simulink model "Rate_Modulation_2"  (R2023a)
settings: Solver=VariableStepAuto  StartTime=0.0  StopTime=100  RelTol=1e-3
model workspace (MAT data in the model file):
  Acc_threshold = Simulink.Parameter
  Acc_threshold.Value = 10
  Acc_threshold.Description = 'minimo valore dell''accelerometro per cui considero paziente in attività'
  Acc_threshold.DataType = 'auto'
  Acc_threshold.Complexity = 'real'
  Acc_threshold.Dimensions = [1 1]
  Activity_response_factor = Simulink.Parameter
  Activity_response_factor.Value = 0.4
  Activity_response_factor.Description = '0<activity response factor<1
    | 
    | max activity setup: activity response factor=1, cioè si raggiunge solo alla massima capacità del sensore il valore MSR_TOP
    | '
  Activity_response_factor.DataType = 'auto'
  Activity_response_factor.Complexity = 'real'
  Activity_response_factor.Dimensions = [1 1]
  Baseline = Simulink.Parameter
  Baseline.Value = 144
  Baseline.Description = 'respiratory rate (average:12) * tidal volume (average:12) in the person
    | -> varies depending on height age gender'
  Baseline.DataType = 'auto'
  Baseline.Complexity = 'real'
  Baseline.Dimensions = [1 1]
  LRL = Simulink.Parameter
  LRL.Value = 60
  LRL.Description = 'Lowest Rate Level'
  LRL.DataType = 'auto'
  LRL.Complexity = 'real'
  LRL.Dimensions = [1 1]
  MSR = Simulink.Parameter
  MSR.Value = 150
  MSR.Description = 'Max Stimulated Rate'
  MSR.DataType = 'auto'
  MSR.Complexity = 'real'
  MSR.Dimensions = [1 1]
  MSR_TOP = Simulink.Parameter
  MSR_TOP.Value = 220
  MSR_TOP.Description = 'max msr: quello con cui faccio le curve, non l''effettivo limite
    | 
    | oss: LRL non ha questa distinzione perchè tendenzialmente è sempre lo stesso'
  MSR_TOP.DataType = 'auto'
  MSR_TOP.Complexity = 'real'
  MSR_TOP.Dimensions = [1 1]
  Metabolic_response_factor = Simulink.Parameter
  Metabolic_response_factor.Value = 0.8
  Metabolic_response_factor.Description = '0<Metabolic_response_factor<1
    | 
    | max metabolic setup: Metabolic_response_factor=1, cioè si raggiunge solo alla massima capacità del sensore il valore MSR_TOP
    | '
  Metabolic_response_factor.DataType = 'auto'
  Metabolic_response_factor.Complexity = 'real'
  Metabolic_response_factor.Dimensions = [1 1]
  Plateau = Simulink.Parameter
  Plateau.Value = 90
  Plateau.Description = '90-95'
  Plateau.DataType = 'auto'
  Plateau.Complexity = 'real'
  Plateau.Dimensions = [1 1]
  Rate_modulation_type = Simulink.Parameter
  Rate_modulation_type.Value = 3
  Rate_modulation_type.Description = '1: integrazione1
    | 2: integrazione2
    | 3: solo acc
    | 4: solo mv'
  Rate_modulation_type.DataType = 'auto'
  Rate_modulation_type.Complexity = 'real'
  Rate_modulation_type.Dimensions = [1 1]
  Reaction_time = 10
  VT_BPM = Simulink.Parameter
  VT_BPM.Value = 156
  VT_BPM.Description = 'battiti a cui corrisponde MV threshold dato il response factor detereminato da MSR e LRL
    | con Ventilatory_Threshold = 60 -> 156 (60-220)
    | '
  VT_BPM.DataType = 'auto'
  VT_BPM.Complexity = 'real'
  VT_BPM.Dimensions = [1 1]
  Ventilatory_Threshold = Simulink.Parameter
  Ventilatory_Threshold.Value = 60
  Ventilatory_Threshold.DataType = 'auto'
  Ventilatory_Threshold.Complexity = 'real'
  Ventilatory_Threshold.Dimensions = [1 1]
  Ventilatory_threshold_response = Simulink.Parameter
  Ventilatory_threshold_response.Value = 0.8
  Ventilatory_threshold_response.Description = '1: OFF
    | 0<Ventilatory_threshold_response<1 '
  Ventilatory_threshold_response.DataType = 'auto'
  Ventilatory_threshold_response.Complexity = 'real'
  Ventilatory_threshold_response.Dimensions = [1 1]
undefined symbols (not defined in the file or in its folder): MAX_MV
libraries: SignalEditorBlockLib x1, dspstat3 x1
settings Model: Creator=fican  LastModifiedBy=fican
settings DebuggingCC: UnconnectedInputMsg=warning  UnconnectedOutputMsg=warning  UnconnectedLineMsg=warning
settings ModelReferenceCC: EnableRefExpFcnMdlSchedulingChecks=on
settings RTWCC: DLArmComputeVersion=19.05

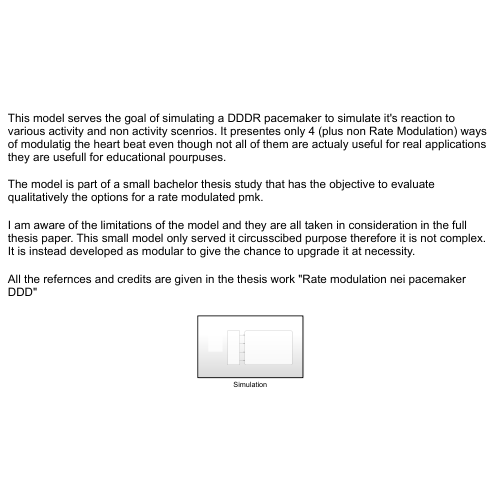
[thumbnail: Simulink's stored preview of the top-level diagram]
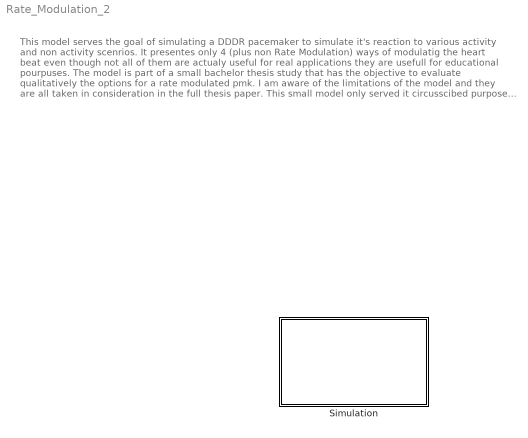
== system Rate_Modulation_2 ==
  note: This model serves the goal of simulating a DDDR pacemaker to simulate it's reaction to various activity and non activity scenrios. It presentes only 4 (plus non Rate Modulation) ways of modulatig the heart beat even though not all of them are actualy useful for real applications they are usefull for educational pourpuses.
      |
      | The model is part of a small bachelor thesis study that has the objective to evaluate qualitatively the options for a rate modulated pmk.
      |
      | I am aware of the limitations of the model and they are all taken in consideration in the full thesis paper. This small model only served it circusscibed purpose therefore it is not complex. It is instead developed as modular to give the chance to upgrade it at necessity.
      |
      | All the refernces and credits are given in the thesis work "Rate modulation nei pacemaker DDD"
  Simulation : Subsystem

== system Rate_Modulation_2/Simulation ==
  note: This stateflow subsystem is the heart of the model
      |
      |
      | sorry for the word play, i had to do it.
  note: This block gives in input simple scenarios created specifally to evaluate the model behaviour in some circustances. It has already a list of some geeric conditions and some limit ones.
      |
      | The only sensors taken for this model are an accelerometer as activity sensor and a minute ventilation as a metabolic sensor.
  Input scenario : SignalEditorBlockLib/Signal Editor  FileName=Scenario2.mat  ActiveScenario=Esercizio  ActiveSignal=Atrium_0  IsBus=off  OutputBusObjectStr=Bus: BusObject  SampleTime=0.001  Interpolate=off  ZeroCross=off  OutputAfterFinalValue=Setting to zero  Unit=inherit  PreserveSignalName=on  ApplySigPropsToAllScenarios=on
  Pacemaker : Stateflow chart  TreatAsAtomicUnit=on
  wires:
  Input scenario/1 -> Pacemaker/1(Atrium)
  Input scenario/3 -> Pacemaker/3(acc_percent)
  Input scenario/2 -> Pacemaker/2(Ventricle)
  Input scenario/4 -> Pacemaker/4(mv_percent)

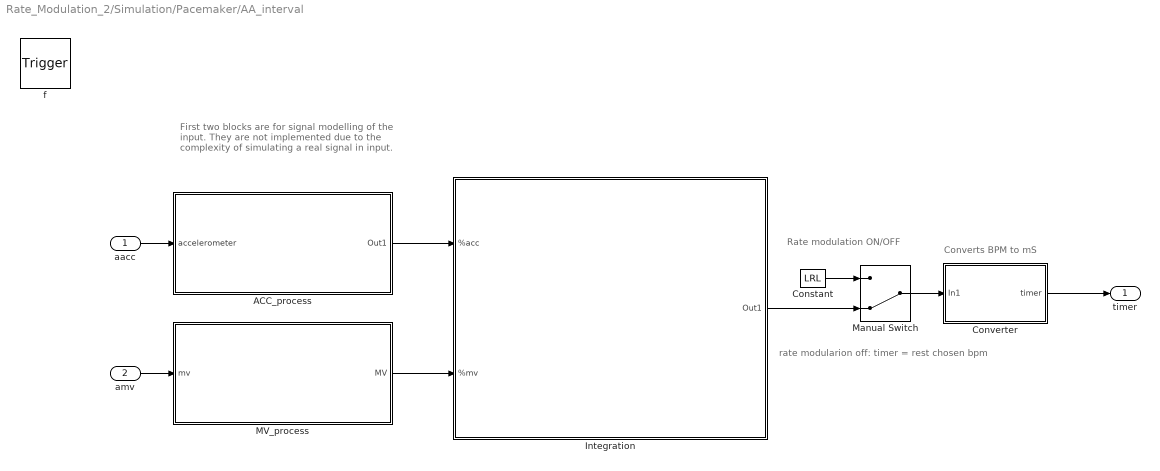
== system Rate_Modulation_2/Simulation/Pacemaker/AA_interval ==
  note: Rate modulation ON/OFF
  note: First two blocks are for signal modelling of the input. They are not implemented due to the complexity of simulating a real signal in input.
  note: Converts BPM to mS
  note: rate modularion off: timer = rest chosen bpm
  aacc : Inport  OutDataTypeStr=double  Unit=1  PortDimensions=1
  amv : Inport  Port=2  OutDataTypeStr=double  Unit=1  PortDimensions=1
  f : TriggerPort  TriggerType=function-call  VariantControl=(inherit)
      settings: CopyFcn=Stateflow.SLINSF.SimulinkMan.removeBlockPreDeleteFcn  PreDeleteFcn=Stateflow.SLINSF.SimulinkMan.unsafePredeleteFcn
  ACC_process : Subsystem
  Constant : Constant  Value=LRL
  Converter : Subsystem
  Integration : Subsystem
  MV_process : Subsystem
  Manual Switch : ManualSwitch  CurrentSetting=0
  timer : Outport
  wires:
  Constant/1 -> Manual Switch/1
  Integration/1(Out1) -> Manual Switch/2
  Converter/1(timer) -> timer/1
  Manual Switch/1 -> Converter/1(In1)
  aacc/1 -> ACC_process/1(accelerometer)
  amv/1 -> MV_process/1(mv)
  ACC_process/1(Out1) -> Integration/1(%acc)
  MV_process/1(MV) -> Integration/2(%mv)

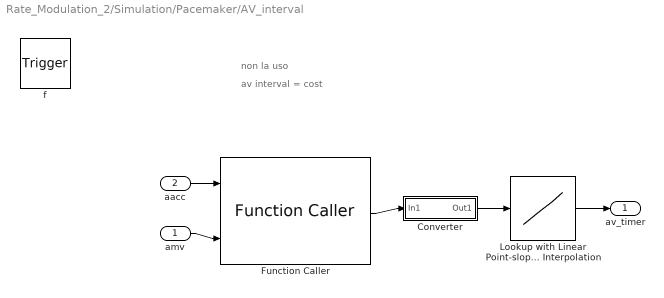
== system Rate_Modulation_2/Simulation/Pacemaker/AV_interval ==
  note: av interval = cost
  note: non la uso
  amv : Inport  OutDataTypeStr=int64  PortDimensions=1
      settings: VarSizeSig=Yes
  aacc : Inport  Port=2  OutDataTypeStr=double  Unit=1  PortDimensions=1
      settings: SignalType=complex
  f : TriggerPort  TriggerType=function-call  VariantControl=(inherit)
      settings: CopyFcn=Stateflow.SLINSF.SimulinkMan.removeBlockPreDeleteFcn  PreDeleteFcn=Stateflow.SLINSF.SimulinkMan.unsafePredeleteFcn
  Converter : Subsystem
  Function Caller : FunctionCaller  FunctionPrototype=timer = AA_interval(aacc,amv)  InputArgumentSpecifications=<Enter example>  OutputArgumentSpecifications=<Enter example>
  Lookup with Linear Point-slope Interpolation : Lookup_n-D  NumberOfTableDimensions=1  BreakpointsForDimension1=[LRL 120]  Table=[175 135]  InternalRulePriority=Speed  RndMeth=Simplest
  av_timer : Outport
  wires:
  aacc/1 -> Function Caller/1
  amv/1 -> Function Caller/2
  Lookup with Linear Point-slope Interpolation/1 -> av_timer/1
  Function Caller/1 -> Converter/1(In1)
  Converter/1(Out1) -> Lookup with Linear Point-slope Interpolation/1

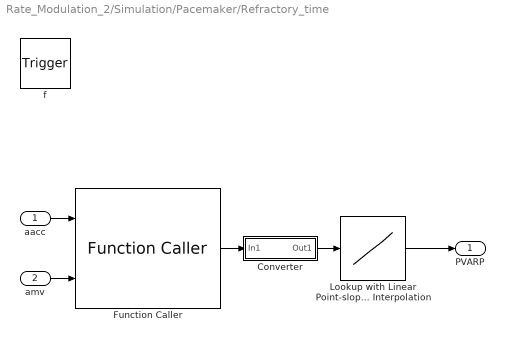
== system Rate_Modulation_2/Simulation/Pacemaker/Refractory_time ==
  aacc : Inport  OutDataTypeStr=double  PortDimensions=1
  amv : Inport  Port=2  OutDataTypeStr=double  PortDimensions=1
  f : TriggerPort  TriggerType=function-call  VariantControl=(inherit)
      settings: CopyFcn=Stateflow.SLINSF.SimulinkMan.removeBlockPreDeleteFcn  PreDeleteFcn=Stateflow.SLINSF.SimulinkMan.unsafePredeleteFcn
  Converter : Subsystem
  Function Caller : FunctionCaller  FunctionPrototype=timer = AA_interval(aacc,amv)  InputArgumentSpecifications=<Enter example>  OutputArgumentSpecifications=<Enter example>
  Lookup with Linear Point-slope Interpolation : Lookup_n-D  NumberOfTableDimensions=1  BreakpointsForDimension1=[LRL 120]  Table=[400 370]  InternalRulePriority=Speed  RndMeth=Simplest
  PVARP : Outport
  wires:
  aacc/1 -> Function Caller/1
  amv/1 -> Function Caller/2
  Function Caller/1 -> Converter/1(In1)
  Converter/1(Out1) -> Lookup with Linear Point-slope Interpolation/1
  Lookup with Linear Point-slope Interpolation/1 -> PVARP/1

== system Rate_Modulation_2/Simulation/Pacemaker/AA_interval/ACC_process ==
  note: The idea here was just to convert the volt signal to a 0-100 value that indicates how much activity is done by the patient. In this model the processing of the signal is not present.
      |
      | It is only present the gain that allows the 'doctor' to regulate the response to activity factor.
      |
      | The simplest way in wich i would have inplemented the signal processing would have been to convert the volt input into a frequency value (considering the smallest period of the oscillatinf signal). This value would have been interpoled beween 0-100 (the actual value input that i'm considering project standing) with the lowest (probably respiratory rate and not zero) and maximum frequency i would have expected from my sensor.
  accelerometer : Inport
  Gain : Gain  Gain=Activity_response_factor
  Out1 : Outport
  wires:
  Gain/1 -> Out1/1
  accelerometer/1 -> Gain/1

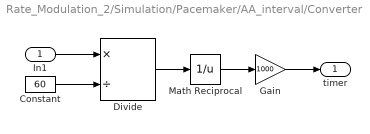
== system Rate_Modulation_2/Simulation/Pacemaker/AA_interval/Converter ==
  In1 : Inport
  Constant : Constant  Value=60
  Divide : Product  Inputs=*/
  Gain : Gain  Gain=1000
  Math Reciprocal : Math  Operator=reciprocal  SignedPower=on
  timer : Outport
  wires:
  In1/1 -> Divide/1
  Constant/1 -> Divide/2
  Divide/1 -> Math Reciprocal/1
  Math Reciprocal/1 -> Gain/1
  Gain/1 -> timer/1

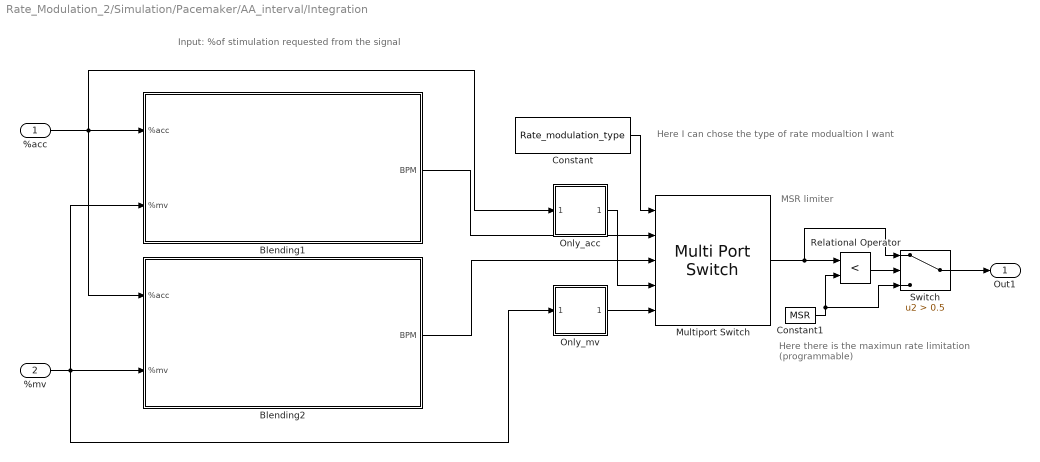
== system Rate_Modulation_2/Simulation/Pacemaker/AA_interval/Integration ==
  note: MSR limiter
  note: Here there is the maximun rate limitation (programmable)
  note: Input: %of stimulation requested from the signal
  note: Here I can chose the type of rate modualtion I want
  %acc : Inport
  %mv : Inport  Port=2
  Blending1 : Subsystem
  Blending2 : Subsystem
  Constant : Constant  Value=Rate_modulation_type
  Constant1 : Constant  Value=MSR
  Multiport Switch : MultiPortSwitch  Inputs=4  DataPortIndices={1,2,3,0}  SaturateOnIntegerOverflow=off  InputSameDT=off
  Only_acc : Subsystem
  Only_mv : Subsystem
  Relational Operator : RelationalOperator  Operator=<  OutDataTypeStr=boolean  RndMeth=Simplest  InputSameDT=off
  Switch : Switch  Criteria=u2 > Threshold  Threshold=0.5  RndMeth=Round  SaturateOnIntegerOverflow=off  InputSameDT=off
  Out1 : Outport
  wires:
  Constant/1 -> Multiport Switch/1
  %acc/1 -> Only_acc/1(%acc), Blending1/1(%acc), Blending2/1(%acc)
  %mv/1 -> Blending2/2(%mv), Only_mv/1(%mv), Blending1/2(%mv)
  Only_acc/1(Out1) -> Multiport Switch/4
  Only_mv/1(Out1) -> Multiport Switch/5
  Blending1/1(BPM) -> Multiport Switch/2
  Blending2/1(BPM) -> Multiport Switch/3
  Multiport Switch/1 -> Switch/1, Relational Operator/1
  Constant1/1 -> Relational Operator/2, Switch/3
  Relational Operator/1 -> Switch/2
  Switch/1 -> Out1/1

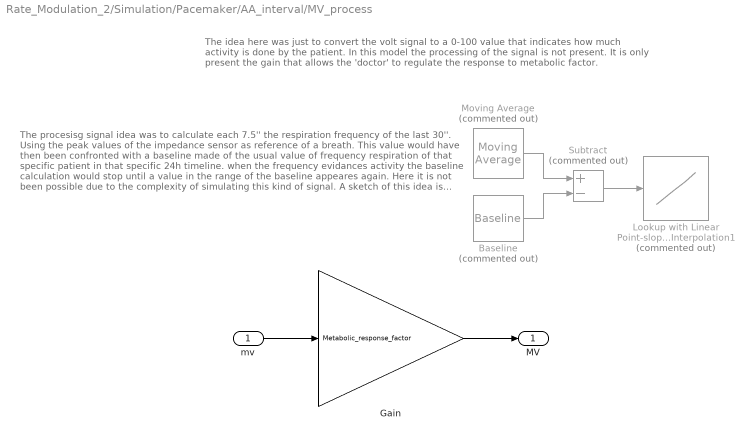
== system Rate_Modulation_2/Simulation/Pacemaker/AA_interval/MV_process ==
  note: The procesisg signal idea was to calculate each 7.5'' the respiration frequency of the last 30''. Using the peak values of the impedance sensor as reference of a breath. This value would have then been confronted with a baseline made of the usual value of frequency respiration of that specific patient in that specific 24h timeline. when the frequency evidances activity the baseline calculation would stop until a value in the range of the baseline appeares again.
      |
      | Here it is not been possible due to the complexity of simulating this kind of signal. A sketch of this idea is present here as a comment.
  note: The idea here was just to convert the volt signal to a 0-100 value that indicates how much activity is done by the patient. In this model the processing of the signal is not present.
      |
      | It is only present the gain that allows the 'doctor' to regulate the response to metabolic factor.
  mv : Inport
  Baseline : Constant  Commented=on  Value=Baseline
  Gain : Gain  Gain=Metabolic_response_factor
  Lookup with Linear Point-slope Interpolation1 : Lookup_n-D  Commented=on  NumberOfTableDimensions=1  BreakpointsForDimension1=[0 MAX_MV]  Table=[0 100]  InternalRulePriority=Speed  RndMeth=Simplest
  Moving Average : dspstat3/Moving Average  Commented=on  Method=Sliding window  ForgettingFactorPort=off  SpecifyWindowLength=on  WindowLength=30  OverlapLength=29  AllowArbitraryInputLength=off  ForgettingFactor=0.9  SimulateUsing=Code generation
  Subtract : Sum  Commented=on  Inputs=+-
  MV : Outport
  wires:
  Baseline/1 -> Subtract/2
  Moving Average/1 -> Subtract/1
  Subtract/1 -> Lookup with Linear Point-slope Interpolation1/1
  mv/1 -> Gain/1
  Gain/1 -> MV/1

== system Rate_Modulation_2/Simulation/Pacemaker/AV_interval/Converter ==
  In1 : Inport
  Gain : Gain  Gain=0.001
  Gain1 : Gain  Gain=60
  Math Reciprocal : Math  Operator=reciprocal  SignedPower=on
  Out1 : Outport
  wires:
  Gain/1 -> Math Reciprocal/1
  In1/1 -> Gain/1
  Math Reciprocal/1 -> Gain1/1
  Gain1/1 -> Out1/1

== system Rate_Modulation_2/Simulation/Pacemaker/Refractory_time/Converter ==
  In1 : Inport
  Gain : Gain  Gain=0,001
  Gain1 : Gain  Gain=60
  Math Reciprocal : Math  Operator=reciprocal  SignedPower=on
  Out1 : Outport
  wires:
  Gain/1 -> Math Reciprocal/1
  In1/1 -> Gain/1
  Math Reciprocal/1 -> Gain1/1
  Gain1/1 -> Out1/1

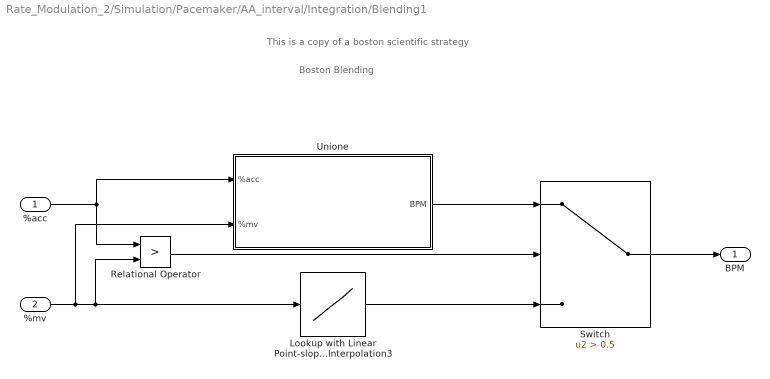
== system Rate_Modulation_2/Simulation/Pacemaker/AA_interval/Integration/Blending1 ==
  note: This is a copy of a boston scientific strategy
  note: Boston Blending
  %acc : Inport
  %mv : Inport  Port=2
  Lookup with Linear Point-slope Interpolation3 : Lookup_n-D  NumberOfTableDimensions=1  BreakpointsForDimension1=[0 100]  Table=[LRL MSR_TOP]  InternalRulePriority=Speed  RndMeth=Simplest
  Relational Operator : RelationalOperator  Operator=>  OutDataTypeStr=boolean  RndMeth=Simplest  InputSameDT=off
  Switch : Switch  Criteria=u2 > Threshold  Threshold=0.5  SaturateOnIntegerOverflow=off  InputSameDT=off
  Unione : Subsystem
  BPM : Outport
  wires:
  %acc/1 -> Unione/1(%acc), Relational Operator/1
  %mv/1 -> Relational Operator/2, Lookup with Linear Point-slope Interpolation3/1, Unione/2(%mv)
  Relational Operator/1 -> Switch/2
  Switch/1 -> BPM/1
  Unione/1(BPM) -> Switch/1
  Lookup with Linear Point-slope Interpolation3/1 -> Switch/3

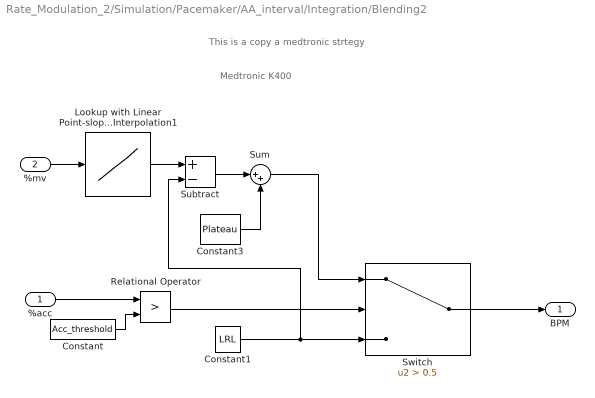
== system Rate_Modulation_2/Simulation/Pacemaker/AA_interval/Integration/Blending2 ==
  note: This is a copy a medtronic strtegy
  note: Medtronic K400
  %acc : Inport
  %mv : Inport  Port=2
  Constant : Constant  Value=Acc_threshold
  Constant1 : Constant  Value=LRL
  Constant3 : Constant  Value=Plateau
  Lookup with Linear Point-slope Interpolation1 : Lookup_n-D  NumberOfTableDimensions=1  BreakpointsForDimension1=[0 100]  Table=[LRL MSR_TOP]  InternalRulePriority=Speed  RndMeth=Simplest
  Relational Operator : RelationalOperator  Operator=>  OutDataTypeStr=boolean  RndMeth=Simplest  InputSameDT=off
  Subtract : Sum  Inputs=+-
  Sum : Sum  Inputs=|++
  Switch : Switch  Criteria=u2 > Threshold  Threshold=0.5  SaturateOnIntegerOverflow=off  InputSameDT=off
  BPM : Outport
  wires:
  %acc/1 -> Relational Operator/1
  Constant/1 -> Relational Operator/2
  Relational Operator/1 -> Switch/2
  Constant1/1 -> Subtract/2, Switch/3
  Lookup with Linear Point-slope Interpolation1/1 -> Subtract/1
  Subtract/1 -> Sum/1
  Constant3/1 -> Sum/2
  %mv/1 -> Lookup with Linear Point-slope Interpolation1/1
  Sum/1 -> Switch/1
  Switch/1 -> BPM/1

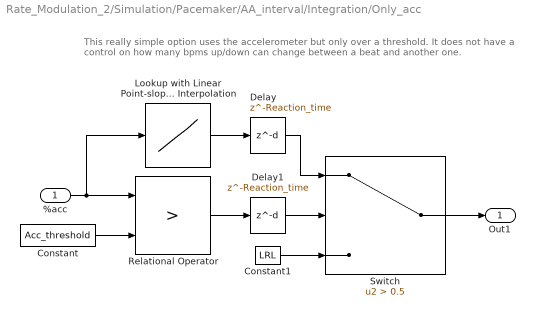
== system Rate_Modulation_2/Simulation/Pacemaker/AA_interval/Integration/Only_acc ==
  note: This really simple option uses the accelerometer but only over a threshold. It does not have a control on how many bpms up/down can change between a beat and another one.
  %acc : Inport
  Constant : Constant  Value=Acc_threshold
  Constant1 : Constant  Value=LRL
  Delay : Delay  DelayLength=Reaction_time
  Delay1 : Delay  DelayLength=Reaction_time
  Lookup with Linear Point-slope Interpolation : Lookup_n-D  NumberOfTableDimensions=1  BreakpointsForDimension1=[Acc_threshold 100+Acc_threshold]  Table=[LRL MSR_TOP]  InternalRulePriority=Speed  RndMeth=Simplest
  Relational Operator : RelationalOperator  Operator=>  OutDataTypeStr=boolean  ZeroCross=off  RndMeth=Simplest  InputSameDT=off
  Switch : Switch  Criteria=u2 > Threshold  Threshold=0.5  OutDataTypeStr=double  SaturateOnIntegerOverflow=off  InputSameDT=off
  Out1 : Outport
  wires:
  Relational Operator/1 -> Delay1/1
  Constant/1 -> Relational Operator/2
  %acc/1 -> Lookup with Linear Point-slope Interpolation/1, Relational Operator/1
  Constant1/1 -> Switch/3
  Delay1/1 -> Switch/2
  Lookup with Linear Point-slope Interpolation/1 -> Delay/1
  Delay/1 -> Switch/1
  Switch/1 -> Out1/1

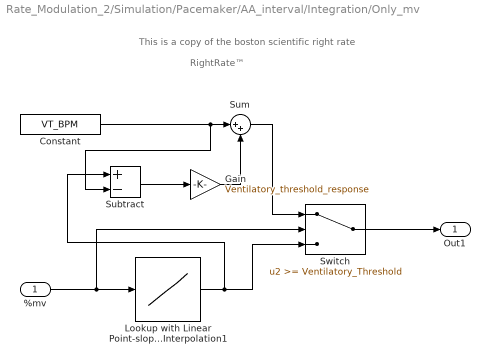
== system Rate_Modulation_2/Simulation/Pacemaker/AA_interval/Integration/Only_mv ==
  note: This is a copy of the boston scientific right rate
  note: RightRate™
  %mv : Inport
  Constant : Constant  Value=VT_BPM
  Gain : Gain  Gain=Ventilatory_threshold_response
  Lookup with Linear Point-slope Interpolation1 : Lookup_n-D  NumberOfTableDimensions=1  BreakpointsForDimension1=[0 100]  Table=[LRL MSR_TOP]  InternalRulePriority=Speed  RndMeth=Simplest
  Subtract : Sum  Inputs=+-
  Sum : Sum  Inputs=|++
  Switch : Switch  Threshold=Ventilatory_Threshold  SaturateOnIntegerOverflow=off  InputSameDT=off
  Out1 : Outport
  wires:
  %mv/1 -> Switch/2, Lookup with Linear Point-slope Interpolation1/1
  Lookup with Linear Point-slope Interpolation1/1 -> Subtract/1, Switch/3
  Switch/1 -> Out1/1
  Constant/1 -> Subtract/2, Sum/1
  Gain/1 -> Sum/2
  Sum/1 -> Switch/1
  Subtract/1 -> Gain/1

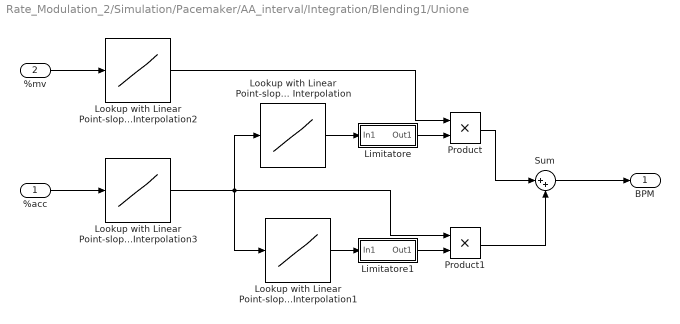
== system Rate_Modulation_2/Simulation/Pacemaker/AA_interval/Integration/Blending1/Unione ==
  %acc : Inport
  %mv : Inport  Port=2
  Limitatore : Subsystem
  Limitatore1 : Subsystem
  Lookup with Linear Point-slope Interpolation : Lookup_n-D  NumberOfTableDimensions=1  BreakpointsForDimension1=[LRL MSR_TOP]  Table=[0.2 0.6]  InternalRulePriority=Speed  RndMeth=Simplest
  Lookup with Linear Point-slope Interpolation1 : Lookup_n-D  NumberOfTableDimensions=1  BreakpointsForDimension1=[LRL MSR_TOP]  Table=[0.8 0.4]  InternalRulePriority=Speed  RndMeth=Simplest
  Lookup with Linear Point-slope Interpolation2 : Lookup_n-D  NumberOfTableDimensions=1  BreakpointsForDimension1=[0 100]  Table=[LRL MSR_TOP]  InternalRulePriority=Speed  RndMeth=Simplest
  Lookup with Linear Point-slope Interpolation3 : Lookup_n-D  NumberOfTableDimensions=1  BreakpointsForDimension1=[0 100]  Table=[LRL MSR_TOP]  InternalRulePriority=Speed  RndMeth=Simplest
  Product : Product
  Product1 : Product
  Sum : Sum  Inputs=|++
  BPM : Outport
  wires:
  %acc/1 -> Lookup with Linear Point-slope Interpolation3/1
  %mv/1 -> Lookup with Linear Point-slope Interpolation2/1
  Product/1 -> Sum/1
  Product1/1 -> Sum/2
  Lookup with Linear Point-slope Interpolation2/1 -> Product/1
  Lookup with Linear Point-slope Interpolation3/1 -> Lookup with Linear Point-slope Interpolation1/1, Product1/1, Lookup with Linear Point-slope Interpolation/1
  Sum/1 -> BPM/1
  Lookup with Linear Point-slope Interpolation/1 -> Limitatore/1(In1)
  Limitatore/1(Out1) -> Product/2
  Limitatore1/1(Out1) -> Product1/2
  Lookup with Linear Point-slope Interpolation1/1 -> Limitatore1/1(In1)

== system Rate_Modulation_2/Simulation/Pacemaker/AA_interval/Integration/Blending1/Unione/Limitatore ==
  In1 : Inport
  Constant : Constant  Value=0.4
  Relational Operator : RelationalOperator  Operator=<  OutDataTypeStr=boolean  RndMeth=Simplest  InputSameDT=off
  Switch : Switch  Criteria=u2 > Threshold  Threshold=0.5  SaturateOnIntegerOverflow=off  InputSameDT=off
  Out1 : Outport
  wires:
  Relational Operator/1 -> Switch/2
  In1/1 -> Switch/1, Relational Operator/1
  Constant/1 -> Switch/3, Relational Operator/2
  Switch/1 -> Out1/1

== system Rate_Modulation_2/Simulation/Pacemaker/AA_interval/Integration/Blending1/Unione/Limitatore1 ==
  In1 : Inport
  Constant : Constant  Value=0.6
  Relational Operator : RelationalOperator  Operator=>  OutDataTypeStr=boolean  RndMeth=Simplest  InputSameDT=off
  Switch : Switch  Criteria=u2 > Threshold  Threshold=0.5  SaturateOnIntegerOverflow=off  InputSameDT=off
  Out1 : Outport
  wires:
  Relational Operator/1 -> Switch/2
  In1/1 -> Switch/1, Relational Operator/1
  Constant/1 -> Switch/3, Relational Operator/2
  Switch/1 -> Out1/1

== stateflow chart Rate_Modulation_2/Simulation/Pacemaker ==
  note: The goal here is to simulate the two chambers and the pacemaker response to their natural behaviour (DDD). A stateflow chart like this is really simple and speakes for itself.
      | For each chaber a period between a beat and the next one is calculated evaluating the patient parameters. The pacemaker will then wait for a spontaneous beat untile the end of that period, when it will give the stimulation (then the beat) by itself.
      |
      | Missing a model of the heart it has not been actually possible to simulate spontaneous beats with rate modulation active. The real heart beat simulation would not be aware of the pacemaker stimulation and 'reset' it's natural timer from there.
  state AtriumLogic [parallel]
    settings: executionOrder=1
    state AtriumSensing
      entry:
      Atrium_beat = 0
      A_sensing =  0
      during:
      Atrium_beat = Stimulate1 (AA_Timer, A_sensing)
      A_sensing =  Atrium
      a_sensing = A_sensing*1000
    state Refractory
      entry:
      Atrium_beat = 0
      A_sensing = 0
    (default) -> AtriumSensing
    AtriumSensing -> AtriumLogic.Refractory : [Atrium_beat == 1]
    AtriumLogic.Refractory -> AtriumSensing : after (250, msec)
        | %dato costante che permette di lavorare anche a 220BPM%
  state Ventricle [parallel]
    settings: executionOrder=3
    state VentricleSensing
      entry:
      Ventricle_beat = 0
      V_sensing = Ventricle
      during:
      Ventricle_beat = Stimulate1 (AV_Timer, V_sensing)
    state Refractory
      entry:
      V_sensing = 0
      Ventricle_beat = 0
    (default) -> VentricleSensing
    VentricleSensing -> Ventricle.Refractory : [Ventricle_beat == 1]
    Ventricle.Refractory -> VentricleSensing : after (100, msec)
  state TriggeredTimer [parallel]
    settings: executionOrder=2
    state AA_timer_working
      entry:
      AA_Timer = AA_interval (acc_percent, mv_percent)
      aa_Timer = AA_interval (acc_percent, mv_percent)
      during:
      AA_Timer = AA_Timer - 1
    state Reset
      entry:
      AA_Timer = 2
    (default) -> AA_timer_working
    AA_timer_working -> TriggeredTimer.Reset : [AA_Timer == 0 || Atrium_beat == 1]
    TriggeredTimer.Reset -> AA_timer_working : after (1, msec)
  state AVTimer [parallel]
    settings: executionOrder=4
    state Reset
      entry:
      AV_Timer = 2
    state AV_Timer_working
      entry:
      AV_Timer = 175 %LRL_value%
      during:
      AV_Timer = AV_Timer -1
    (default) -> AVTimer.Reset
    AV_Timer_working -> AVTimer.Reset : [AV_Timer == 0 || Ventricle_beat == 1]
    AVTimer.Reset -> AV_Timer_working : [Atrium_beat == 1]
  state beat = Stimulate1 (timer, sensing) [function]
    (default) -> (junction 45) : {beat = 0}
    (junction 45) -> (junction 51) [order 1] : [timer > 0 ]
    (junction 51) -> (junction 73) [order 2] : {beat= 0}
    (junction 51) -> (junction 53) [order 1] : [sensing > 1.25]
    (junction 45) -> (junction 53) [order 2] : [timer <= 0]
    (junction 53) -> (junction 149) : {beat=1}
  state timer = AA_interval(aacc,amv) [function]
  state av_timer = AV_interval(amv,aacc) [function] [commented out]
  note: This two 'timer' funcions are the beat(s) period timer. They regulate the increase/decrese of the beat(s) frequency. Obvously they only intervene to regulate natulal heart beat for higer frequency requestes.
      | When rate modulation is on this two timers are in charge of stating the right beat frequency.
      |
      | For time and semplicity reasons only the Atrium-Atrium timer is been fully implemented. For the Atrium-Ventricle timer a fixed time is used.
  note: This block should serve the purpose of simulating the behaviour of the pmk of going in refractory mode just after the beat(s) for each chamber sensed.
      | It is not been implemented for time reasons.
  state PVARP = Refractory_time(aacc,amv) [function] [commented out]
  data: timer function_input; sensing function_input; beat function_output; timer function_output; aacc function_input double size=1; amv function_input double size=1; av_timer function_output double size=1; amv function_input double size=1; aacc function_input double size=1; aacc function_input double size=1; amv function_input double size=1; PVARP function_output double size=1; Atrium input; A_sensing local; AA_Timer local; V_sensing local; Ventricle input; AV_Timer local; Atrium_beat local Simulink.NumericType size=1; Ventricle_beat local; acc_percent input; mv_percent input; aa_Timer local; a_sensing local
